simulink model "Lab1"  (R2018a)
settings: Solver=VariableStepAuto  StartTime=0.0  StopTime=8  RelTol=1e-3
libraries: simulink x3
settings Model: Creator=Ahmed Eldokmak  LastModifiedBy=Ahmed Eldokmak

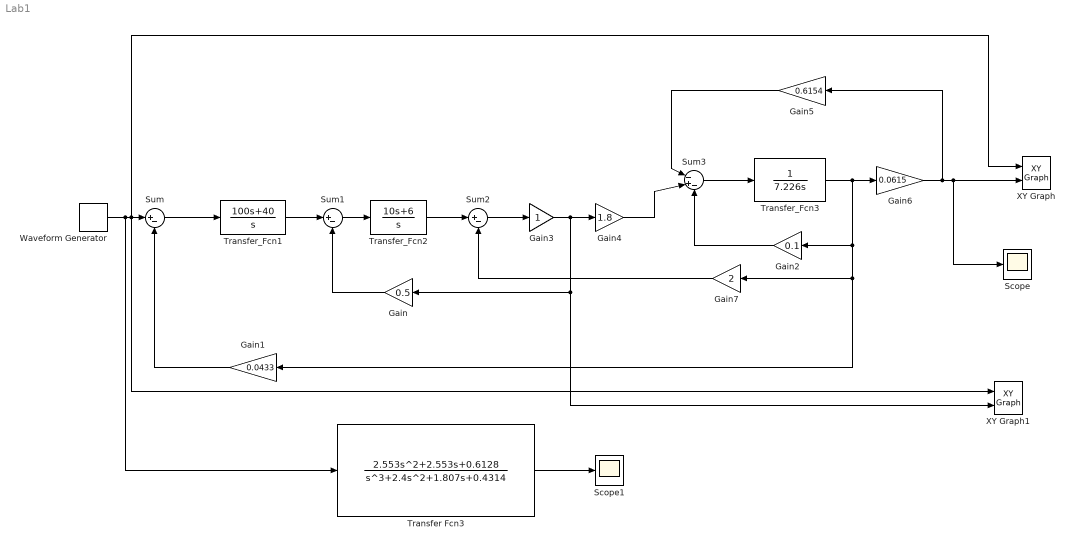
== system Lab1 ==
  Gain : Gain  Gain=0.5
  Gain1 : Gain  Gain=0.0433
  Gain2 : Gain  Gain=0.1
  Gain3 : Gain
  Gain4 : Gain  Gain=1.8
  Gain5 : Gain  Gain=0.6154
  Gain6 : Gain  Gain=0.0615
  Gain7 : Gain  Gain=2
  Scope : Scope
  Scope1 : Scope
  Sum : Sum  Inputs=|+-
  Sum1 : Sum  Inputs=|+-
  Sum2 : Sum  Inputs=|+-
  Sum3 : Sum  Inputs=|-+-
  Transfer Fcn3 : TransferFcn  Numerator=[0 2.553 2.553 0.6128]  Denominator=[1 2.4 1.807 0.4314]
  Transfer_Fcn1 : TransferFcn  Numerator=[100 40]  Denominator=[1 0]
  Transfer_Fcn2 : TransferFcn  Numerator=[10 6]  Denominator=[1 0]
  Transfer_Fcn3 : TransferFcn  Numerator=[0 1]  Denominator=[7.226 0]
  Waveform Generator : simulink/Sources/Waveform Generator  OutMin=[]  OutMax=[]  OutDataTypeStr=double  SelectedSignal=1  Signals=Square('Amplitude',5,'Frequency',5,'Phase',0,'DutyCycle',80)#step('StepTime',0,'InitialValue',0,'FinalValue',1)  BlockNames=MultiportSwitch_c959eabd123a4e3#MultiportSwitch_fbd4f80a687d48a  SampleTime=0.1
      settings: SourceProductName=Simulink
  XY Graph : simulink/Sinks/XY Graph  xmin=-10  xmax=12  ymin=0  ymax=3  st=8
  XY Graph1 : simulink/Sinks/XY Graph  xmin=-10  xmax=10  ymin=700  ymax=1000  st=8
  wires:
  Sum/1 -> Transfer_Fcn1/1
  Sum1/1 -> Transfer_Fcn2/1
  Transfer_Fcn1/1 -> Sum1/1
  Transfer_Fcn2/1 -> Sum2/1
  Gain/1 -> Sum1/2
  Gain1/1 -> Sum/2
  Sum2/1 -> Gain3/1
  Gain4/1 -> Sum3/2
  Sum3/1 -> Transfer_Fcn3/1
  Transfer_Fcn3/1 -> Gain1/1, Gain7/1, Gain2/1, Gain6/1
  Gain2/1 -> Sum3/3
  Gain5/1 -> Sum3/1
  Gain6/1 -> Gain5/1, Scope/1, XY Graph/2
  Gain7/1 -> Sum2/2
  Waveform Generator/1 -> Transfer Fcn3/1, XY Graph1/1, XY Graph/1, Sum/1
  Transfer Fcn3/1 -> Scope1/1
  Gain3/1 -> XY Graph1/2, Gain/1, Gain4/1
